simulink model "Model_vertical_lqr_2016a"  (R2016a)
settings: Solver=ode4  StartTime=0.0  StopTime=25  FixedStep=1e-3  RelTol=1e-3
values from neighbouring files (symbols this model uses):
  a = moment(pwm==0)/-sin(-0.5223)    [Helicopter_main_test.m]    (also in Lin_simulink_test.mat = -0.306762334307; sageno_opt.m = 1)
  alpha_0 = parameters(3)    [Helicopter_main_test.m]    (also in Lin_simulink_test.mat = -0.522258173088)
  f_v = parameters(2)    [Helicopter_main_test.m]
  I_v = lsqnonlin(cel, I_v, 0,[],options)    [Helicopter_main_test.m]
  J_v = parameters(1)    [Helicopter_main_test.m]
  K_lqr = lqr(lin_A, lin_B, Q, R, N)    [Helicopter_main_test.m]
  L = place(lin_A.', lin_C.', lambda).'    [Helicopter_main_test.m]    (also in sageno_opt.m = length(output))
  lin_A = [0 1 0;     a/J_v*cos(lin_alpha_v-alpha_0) -f_v/J_v polyval(lin_M_V_diff, lin_w_v)/J_v;     0 0 -polyval(lin_U_V_diff, lin_w_v)/I_v]    [Helicopter_main_test.m]
  lin_alpha_v = 0    [Helicopter_main_test.m]
  lin_B = [0; 0; 1/I_v]    [Helicopter_main_test.m]
  lin_C = [1 0 0]    [Helicopter_main_test.m]
  lin_u_v = polyval(wsp_U_V, lin_w_v)    [Helicopter_main_test.m]
  lin_velocity_v = 0    [Helicopter_main_test.m]
  lin_w_v = real(lin_w_v(lin_w_v>-330 & lin_w_v<300 & imag(lin_w_v)==0))    [Helicopter_main_test.m]
  wsp_M_V = polyfit(v, moment, 5)    [Helicopter_main_test.m]    (also in Lin_simulink_test.mat = [-2.51456949125e-14 2.95925329869e-12 8.13117134031e-09 5.04)
  wsp_U_V = polyfit(pred,PWM,5)    [Helicopter_main_test.m]    (also in Lin_simulink_test.mat = [-7.44181518745e-14 1.363108664e-11 2.62321306545e-08 -6.605)
settings Model: Creator=Student  LastModifiedBy=Maciek
settings DataIOCC: LimitDataPoints=on  SaveFormat=Array
settings HardwareCC: ProdBitPerPointer=32  ProdLargestAtomicFloat=None  ProdIntDivRoundTo=Undefined  ProdEndianess=Unspecified  ProdWordSize=32  ProdHWDeviceType=32-bit Generic
settings ModelReferenceCC: PropagateSignalLabelsOutOfModel=off

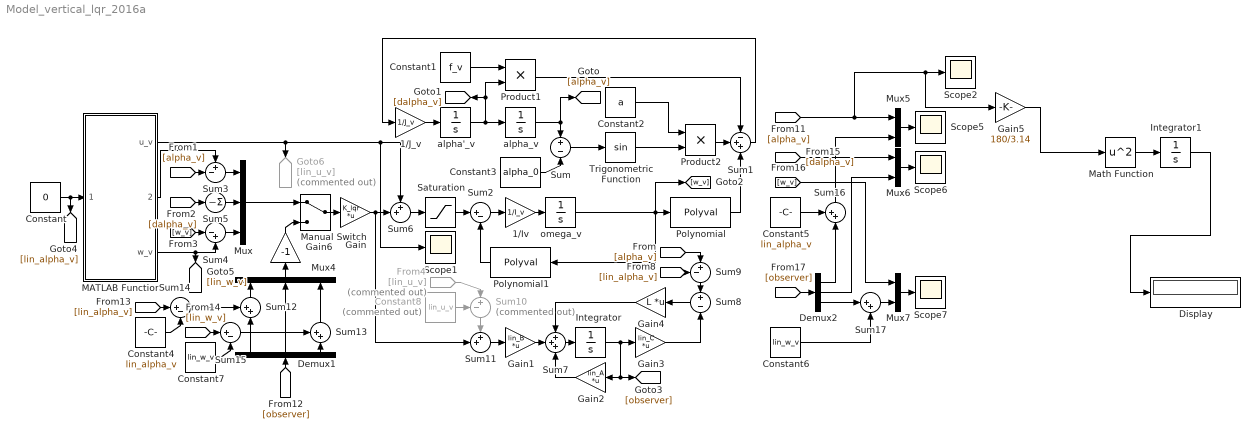
== system Model_vertical_lqr_2016a ==
  1/Iv : Gain  Gain=1/I_v
  1/J_v : Gain  Gain=1/J_v
  Constant : Constant  Value=0
  Constant1 : Constant  Value=f_v
  Constant2 : Constant  Value=a
  Constant3 : Constant  Value=alpha_0
  Constant4 : Constant  Value=lin_alpha_v
  Constant5 : Constant  Value=lin_alpha_v
  Constant6 : Constant  Value=lin_w_v
  Constant7 : Constant  Value=lin_w_v
  Constant8 : Constant  Commented=on  Value=lin_u_v
  Demux1 : Demux  Outputs=3
  Demux2 : Demux  Outputs=3
  Display : Display
  From4 : From  Commented=on  GotoTag=lin_u_v
  Gain : Gain  Gain=K_lqr  Multiplication=Matrix(K*u)
  Gain1 : Gain  Gain=lin_B  Multiplication=Matrix(K*u)
  Gain2 : Gain  Gain=lin_A  Multiplication=Matrix(K*u)
  Gain3 : Gain  Gain=lin_C  Multiplication=Matrix(K*u)
  Gain4 : Gain  Gain=L  Multiplication=Matrix(K*u)
  Gain5 : Gain  Gain=180/3.14
  Gain6 : Gain  Gain=-1
  Goto6 : Goto  Commented=on  GotoTag=lin_u_v
  Integrator : Integrator  InitialCondition=[0;0;0]
  Integrator1 : Integrator
  MATLAB Function : MATLAB Function  TreatAsAtomicUnit=on
  Manual Switch : ManualSwitch
  Math Function : Math  Operator=square  SaturateOnIntegerOverflow=on
  Mux : Mux  Inputs=3
  Mux4 : Mux  Inputs=3
  Mux5 : Mux  Inputs=2
  Mux6 : Mux  Inputs=2
  Mux7 : Mux  Inputs=2
  Polynomial : Polyval  Coefs=wsp_M_V
  Polynomial1 : Polyval  Coefs=wsp_U_V
  Product1 : Product
  Product2 : Product
  Saturation : Saturate  UpperLimit=1  LowerLimit=-1
  Scope{1..2,5..7} (5 alike) : Scope
  Sum : Sum  Inputs=+|-
  Sum1 : Sum  Inputs=-++
  Sum10 : Sum  Commented=on  Inputs=-+|
  Sum{6,11..13,16} (5 alike) : Sum  Inputs=++|
  Sum14 : Sum  Inputs=|+-
  Sum15 : Sum  Inputs=|+-
  Sum17 : Sum  Inputs=|++
  Sum2 : Sum  Inputs=|+-
  Sum3 : Sum  Inputs=+-|
  Sum4 : Sum  Inputs=|-+
  Sum5 : Sum  Inputs=|-|
  Sum7 : Sum  Inputs=+++
  Sum8 : Sum  Inputs=+|-
  Sum9 : Sum  Inputs=-+|
  Trigonometric Function : Trigonometry
  alpha'_v : Integrator  InitialCondition=lin_velocity_v
  alpha_v : Integrator  InitialCondition=lin_alpha_v+alpha_0
  omega_v : Integrator  InitialCondition=lin_w_v
  wires:
  omega_v/1 -> [w_v], Polynomial1/1, Polynomial/1
  Product2/1 -> Sum1/2
  Sum2/1 -> 1/Iv/1
  Sum/1 -> Trigonometric Function/1
  Constant3/1 -> Sum/2
  Constant1/1 -> Product1/1
  alpha_v/1 -> [alpha_v], Sum/1
  Constant2/1 -> Product2/1
  Polynomial/1 -> Sum1/3
  Sum1/1 -> 1/J_v/1
  Product1/1 -> Sum1/1
  1/J_v/1 -> alpha'_v/1
  alpha'_v/1 -> [dalpha_v], Product1/2, alpha_v/1
  Trigonometric Function/1 -> Product2/2
  Polynomial1/1 -> Sum2/2
  1/Iv/1 -> omega_v/1
  [alpha_v] -> Sum9/2
  [alpha_v] -> Sum3/2
  Sum3/1 -> Mux/1
  MATLAB Function/2(alpha_v) -> Sum3/1
  Sum4/1 -> Mux/3
  [w_v] -> Sum4/1
  MATLAB Function/3(w_v) -> [lin_w_v], Sum4/2
  [dalpha_v] -> Sum5/1
  Sum5/1 -> Mux/2
  MATLAB Function/1(u_v) -> Goto6/1, Scope1/1, Sum6/1
  Sum6/1 -> Saturation/1
  Saturation/1 -> Sum2/1
  Gain1/1 -> Sum7/2
  Sum7/1 -> Integrator/1
  Gain2/1 -> Sum7/3
  Integrator/1 -> Gain3/1, [observer], Gain2/1
  Gain3/1 -> Sum8/2
  Sum8/1 -> Gain4/1
  Gain4/1 -> Sum7/1
  Gain/1 -> Sum11/2, Sum6/2
  Constant/1 -> [lin_alpha_v], MATLAB Function/1("alpha_v ")
  Sum9/1 -> Sum8/1
  [lin_alpha_v] -> Sum9/1
  Manual Switch/1 -> Gain/1
  Mux/1 -> Manual Switch/1
  Gain6/1 -> Manual Switch/2
  Sum13/1 -> Mux4/3
  Mux4/1 -> Gain6/1
  Sum12/1 -> Mux4/1
  [observer] -> Demux1/1
  Demux1/1 -> Sum12/2
  Demux1/2 -> Mux4/2
  Demux1/3 -> Sum13/2
  Sum14/1 -> Sum12/1
  Sum15/1 -> Sum13/1
  Constant7/1 -> Sum15/2
  [lin_alpha_v] -> Sum14/1
  [lin_w_v] -> Sum15/1
  Constant4/1 -> Sum14/2
  [dalpha_v] -> Mux6/1
  Sum16/1 -> Mux5/2
  Mux7/1 -> Scope7/1
  Demux2/3 -> Sum17/1
  Mux5/1 -> Scope5/1
  Sum17/1 -> Mux7/2
  Mux6/1 -> Scope6/1
  [observer] -> Demux2/1
  [w_v] -> Mux7/1
  Demux2/2 -> Mux6/2
  Constant5/1 -> Sum16/1
  [alpha_v] -> Gain5/1, Scope2/1, Mux5/1
  Sum11/1 -> Gain1/1
  Sum10/1 -> Sum11/1
  From4/1 -> Sum10/2
  Constant8/1 -> Sum10/1
  Demux2/1 -> Sum16/2
  Constant6/1 -> Sum17/2
  Math Function/1 -> Integrator1/1
  Integrator1/1 -> Display/1
  Gain5/1 -> Math Function/1

== matlab function Model_vertical_lqr_2016a/MATLAB Function ==
  data: u_v output double size=1 [0..1]; alpha_v input; alpha_v output; w_v output double size=1
function [u_v, alpha_v, w_v] = Lin(alpha_v)

const = load('Lin_simulink_test.mat');

w_v = roots(const.wsp_M_V+[zeros(1,length(const.wsp_M_V)-1) const.a*sin(alpha_v-const.alpha_0)]);
w_v = real(w_v(w_v>-350 & w_v<350 & imag(w_v)==0));
w_v = w_v(1);
u_v = polyval(const.wsp_U_V, w_v);
u_v = u_v(1);
